simulink library "AP_YawController"  (R2024a)
settings: Solver=VariableStepAuto  StartTime=0.0  StopTime=10.0  RelTol=1e-3
undefined symbols (not defined in the file): DiscIntNeverNeededParam, RLL_Freq, YAW2SRV_DAMP, YAW2SRV_INT, YAW2SRV_RLL, YAW2SRV_SLIP, YAW_Freq, YAW_RATE_D, YAW_RATE_ENABLE, YAW_RATE_I, YAW_RATE_P
libraries: simulink_extras x2, ArdupilotFunctions x1
settings Model: Creator=igmso  LastModifiedBy=igmso

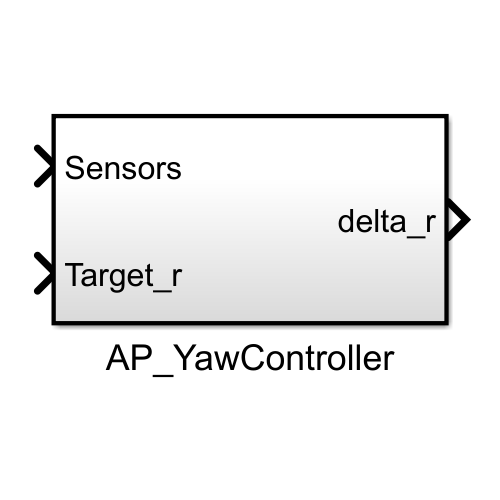
[thumbnail: Simulink's stored preview of the top-level diagram]
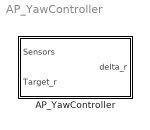
== system AP_YawController ==
  AP_YawController : Subsystem  TreatAsAtomicUnit=on  SystemSampleTime=1/RLL_Freq

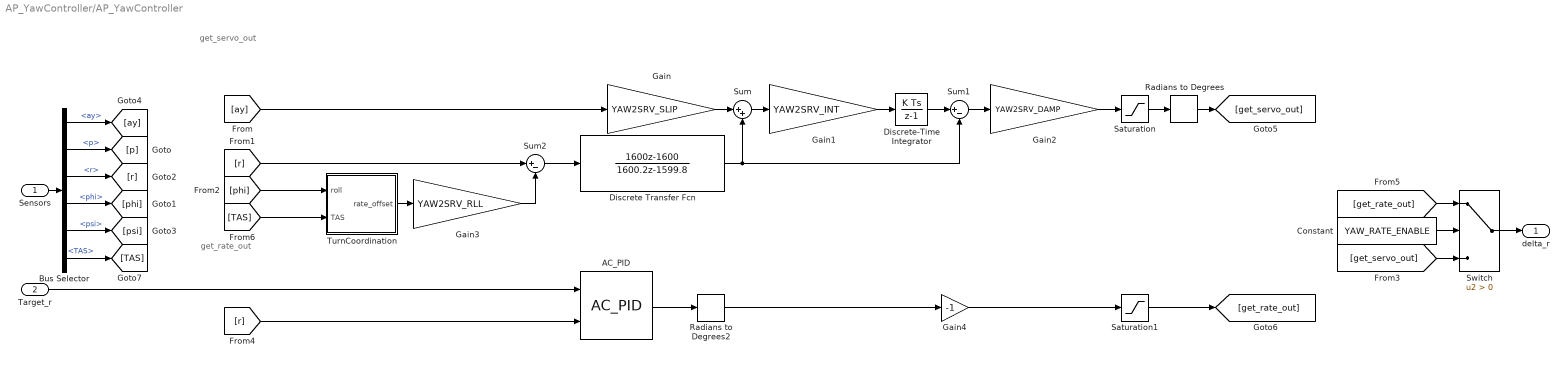
== system AP_YawController/AP_YawController ==
  note: get_servo_out
  note: get_rate_out
  Sensors : Inport
  Target_r : Inport  Port=2  SampleTime=1/YAW_Freq
  AC_PID : ArdupilotFunctions/AC_PID  P=YAW_RATE_P  I=YAW_RATE_I  D=YAW_RATE_D  FF=YAW_RATE_FF  D_FF=YAW_RATE_D_FF  FLTD=YAW_RATE_FLTD  FLTE=YAW_RATE_FLTE  FLTT=YAW_RATE_FLTT  IMAX=YAW_RATE_IMAX  ControlFreq=YAW_Freq
  Bus Selector : BusSelector  OutputSignals=ay,p,r,phi,psi,TAS
  Constant : Constant  Value=YAW_RATE_ENABLE  SampleTime=1/YAW_Freq
  Discrete Transfer Fcn : DiscreteTransferFcn  Numerator=[1600 -1600]  Denominator=[1600.2 -1599.8]
  Discrete-Time Integrator : DiscreteIntegrator  SampleTime=-1  ICPrevOutput=DiscIntNeverNeededParam  ICPrevScaledInput=DiscIntNeverNeededParam
  Gain : Gain  Gain=YAW2SRV_SLIP
  Gain1 : Gain  Gain=YAW2SRV_INT
  Gain2 : Gain  Gain=YAW2SRV_DAMP
  Gain3 : Gain  Gain=YAW2SRV_RLL
  Gain4 : Gain  Gain=-1
  Radians to Degrees : simulink_extras/Transformations/Radians to Degrees
  Radians to Degrees2 : simulink_extras/Transformations/Radians to Degrees
  Saturation : Saturate  UpperLimit=45  LowerLimit=-45
  Saturation1 : Saturate  UpperLimit=45  LowerLimit=-45
  Sum : Sum  Inputs=|++
  Sum1 : Sum  Inputs=|+-
  Sum2 : Sum  Inputs=|+-
  Switch : Switch  Criteria=u2 > Threshold  SaturateOnIntegerOverflow=off  InputSameDT=off
  TurnCoordination : Subsystem
  delta_r : Outport
  wires:
  Saturation1/1 -> [get_rate_out]
  AC_PID/1 -> Radians to Degrees2/1
  Gain4/1 -> Saturation1/1
  Radians to Degrees/1 -> [get_servo_out]
  [phi] -> TurnCoordination/1(roll)
  Saturation/1 -> Radians to Degrees/1
  [r] -> Sum2/1
  [TAS] -> TurnCoordination/2(TAS)
  Bus Selector/6 -> [TAS]  "<TAS>"
  TurnCoordination/1(rate_offset) -> Gain3/1
  [get_rate_out] -> Switch/1
  Radians to Degrees2/1 -> Gain4/1
  [r] -> AC_PID/2
  Target_r/1 -> AC_PID/1
  Constant/1 -> Switch/2
  Switch/1 -> delta_r/1
  [get_servo_out] -> Switch/3
  Gain3/1 -> Sum2/2
  Discrete Transfer Fcn/1 -> Sum1/2, Sum/2
  Sum2/1 -> Discrete Transfer Fcn/1
  Gain2/1 -> Saturation/1
  Sum1/1 -> Gain2/1
  Discrete-Time Integrator/1 -> Sum1/1
  Gain1/1 -> Discrete-Time Integrator/1
  Sum/1 -> Gain1/1
  Gain/1 -> Sum/1
  [ay] -> Gain/1
  Bus Selector/5 -> [psi]  "<psi>"
  Bus Selector/4 -> [phi]  "<phi>"
  Bus Selector/3 -> [r]  "<r>"
  Bus Selector/2 -> [p]  "<p>"
  Bus Selector/1 -> [ay]  "<ay>"
  Sensors/1 -> Bus Selector/1

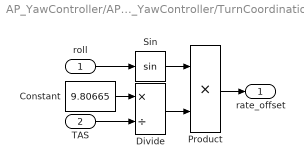
== system AP_YawController/AP_YawController/TurnCoordination ==
  roll : Inport
  TAS : Inport  Port=2
  Constant : Constant  Value=9.80665  SampleTime=1/YAW_Freq
  Divide : Product  Inputs=*/
  Product : Product
  Sin : Trigonometry
  rate_offset : Outport
  wires:
  Product/1 -> rate_offset/1
  Divide/1 -> Product/2
  Sin/1 -> Product/1
  roll/1 -> Sin/1
  TAS/1 -> Divide/2
  Constant/1 -> Divide/1
